simulink model "linearmay19"  (R2021b)
settings: Solver=VariableStepAuto  StartTime=0.0  StopTime=5  RelTol=1e-3
values from neighbouring files (symbols this model uses):
  A0 = finda(l1,l2)    [main.m]
  B0 = findb(l1,l2)    [main.m]
  C0 = findc(l1,l2)    [main.m]
  D0 = findd(l1,l2)    [main.m]
libraries: simulink_extras x2
settings Model: Creator=LEE  LastModifiedBy=LEE

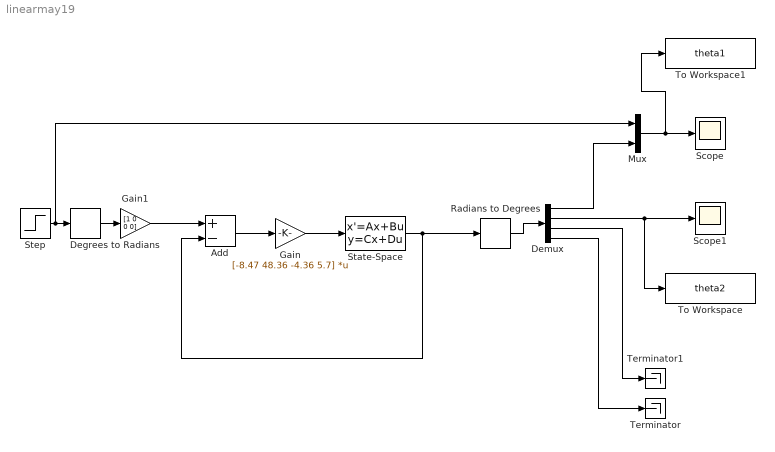
== system linearmay19 ==
  Add : Sum  Inputs=+-
  Degrees to Radians : simulink_extras/Transformations/Degrees to Radians
  Demux : Demux
  Gain : Gain  Gain=[-8.47 48.36 -4.36 5.7]  Multiplication=Matrix(K*u)
  Gain1 : Gain  Gain=[1 0 0 0]
  Mux : Mux  Inputs=2
  Radians to Degrees : simulink_extras/Transformations/Radians to Degrees
  Scope : Scope
  Scope1 : Scope
  State-Space : StateSpace  A=A0  B=B0  C=C0  D=D0  InitialCondition=[0 pi 0 0]
  Step : Step  After=0  SampleTime=0
  Terminator : Terminator
  Terminator1 : Terminator
  To Workspace : ToWorkspace  VariableName=theta2  SampleTime=-1
  To Workspace1 : ToWorkspace  VariableName=theta1  SampleTime=-1
  wires:
  Step/1 -> Mux/1, Degrees to Radians/1
  Degrees to Radians/1 -> Gain1/1
  Add/1 -> Gain/1
  Gain1/1 -> Add/1
  Gain/1 -> State-Space/1
  State-Space/1 -> Add/2, Radians to Degrees/1
  Demux/4 -> Terminator/1
  Demux/3 -> Terminator1/1
  Radians to Degrees/1 -> Demux/1
  Mux/1 -> To Workspace1/1, Scope/1
  Demux/1 -> Mux/2
  Demux/2 -> Scope1/1, To Workspace/1
